simulink model "optimTRIAD"  (R2019a)
settings: Solver=VariableStepAuto  StartTime=0.0  StopTime=10.0  RelTol=1e-3
libraries: vrlib x8, dspstat3 x2, sharedtransform x1, aerolibutil x1
settings Model: Creator=Owner  LastModifiedBy=Owner

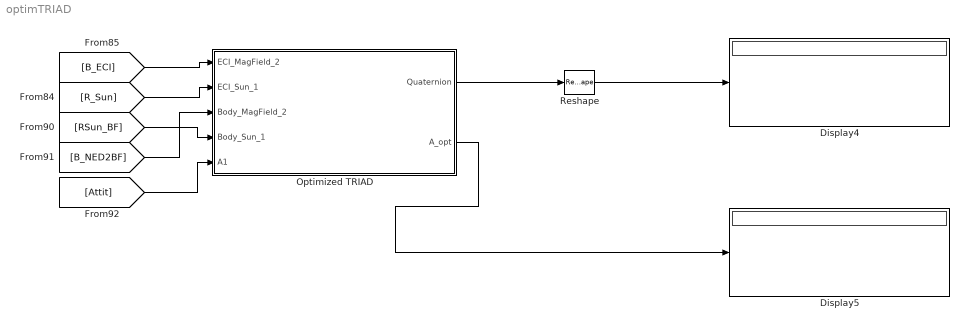
== system optimTRIAD ==
  Display4 : Display
  Display5 : Display
  "Optimized TRIAD " : Subsystem
  Reshape : Reshape  OutputDimensionality=Column vector (2-D)
  wires:
  [RSun_BF] -> "Optimized TRIAD "/4(Body_Sun_1)
  [Attit] -> "Optimized TRIAD "/5(A1)
  [B_NED2BF] -> "Optimized TRIAD "/3(Body_MagField_2)
  "Optimized TRIAD "/1(Quaternion) -> Reshape/1
  [B_ECI] -> "Optimized TRIAD "/1(ECI_MagField_2)
  [R_Sun] -> "Optimized TRIAD "/2(ECI_Sun_1)
  "Optimized TRIAD "/2(A_opt) -> Display5/1
  Reshape/1 -> Display4/1

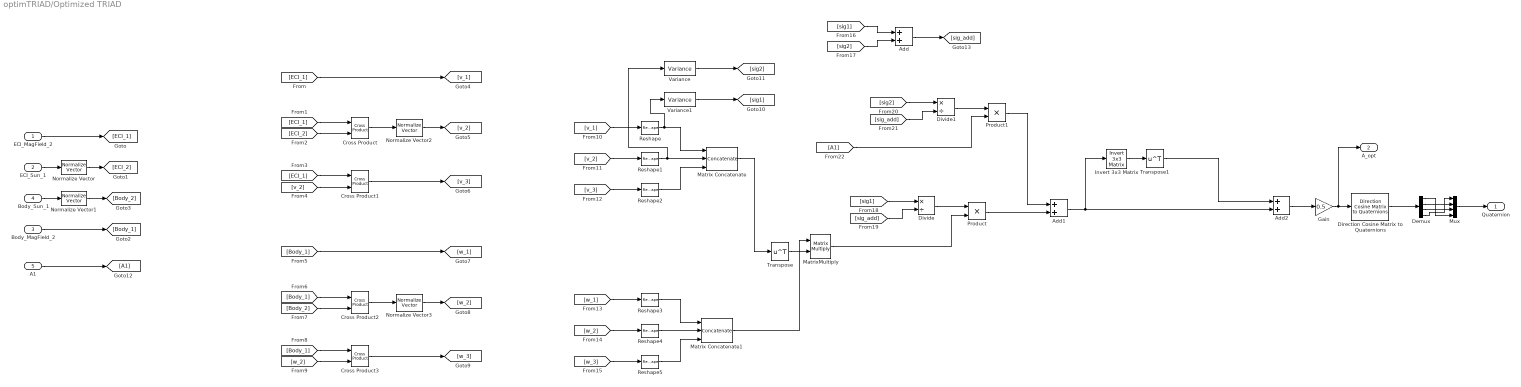
== system optimTRIAD/Optimized TRIAD  ==
  ECI_MagField_2 : Inport
  ECI_Sun_1 : Inport  Port=2
  Body_MagField_2 : Inport  Port=3
  Body_Sun_1 : Inport  Port=4
  A1 : Inport  Port=5
  Add : Sum
  Add1 : Sum
  Add2 : Sum
  Cross Product{,1..3} (4 alike) : vrlib/Utilities/Cross Product
  Demux : Demux
  Direction Cosine Matrix to Quaternions : sharedtransform/Direction Cosine Matrix  to Quaternions  aMode=0  action=None  tolerance=eps(2)
      settings: SourceProductBaseCode=AE,PW,MT,UV,VE,VP
  Divide : Product  Inputs=*/
  Divide1 : Product  Inputs=*/
  Gain : Gain  Gain=0.5
  Invert 3x3 Matrix : aerolibutil/Invert  3x3 Matrix
  Matrix Concatenate : Concatenate  NumInputs=3  Mode=Multidimensional array  ConcatenateDimension=2
  Matrix Concatenate1 : Concatenate  NumInputs=3  Mode=Multidimensional array  ConcatenateDimension=2
  MatrixMultiply : Product  Multiplication=Matrix(*)
  Mux : Mux
  Normalize Vector{,1..3} (4 alike) : vrlib/Utilities/Normalize Vector  maxzero=0
  Product : Product
  Product1 : Product
  Reshape{,1..5} (6 alike) : Reshape  OutputDimensionality=Column vector (2-D)
  Transpose : Math  Operator=transpose  SaturateOnIntegerOverflow=on
  Transpose1 : Math  Operator=transpose  SaturateOnIntegerOverflow=on
  Variance : dspstat3/Variance  run=off  InputProcessing=Columns as channels (frame based)  reset_popup=None  directionMode=Each column  dimension=1  roiEnable=off  roiType=Rectangles  roiPortion=Entire ROI  roiOutput=Individual statistics for each ROI  roiFlag=off  roundingMode=Floor  overflowMode=off
      settings: SourceProductName=DSP System Toolbox
  Variance1 : dspstat3/Variance  run=off  InputProcessing=Columns as channels (frame based)  reset_popup=None  directionMode=Each column  dimension=1  roiEnable=off  roiType=Rectangles  roiPortion=Entire ROI  roiOutput=Individual statistics for each ROI  roiFlag=off  roundingMode=Floor  overflowMode=off
      settings: SourceProductName=DSP System Toolbox
  Quaternion : Outport  VectorParamsAs1DForOutWhenUnconnected=on
  A_opt : Outport  Port=2  VectorParamsAs1DForOutWhenUnconnected=on
  wires:
  Cross Product/1 -> Normalize Vector2/1
  [ECI_1] -> Cross Product1/1
  Reshape2/1 -> Matrix Concatenate/3
  Cross Product3/1 -> [w_3]
  [ECI_1] -> [v_1]
  [w_1] -> Reshape3/1
  Body_Sun_1/1 -> Normalize Vector1/1
  [Body_1] -> Cross Product2/1
  [ECI_1] -> Cross Product/1
  Normalize Vector3/1 -> [w_2]
  Cross Product2/1 -> Normalize Vector3/1
  [Body_1] -> Cross Product3/1
  Cross Product1/1 -> [v_3]
  Normalize Vector2/1 -> [v_2]
  [ECI_2] -> Cross Product/2
  Reshape3/1 -> Matrix Concatenate1/1
  [v_2] -> Cross Product1/2
  [Body_1] -> [w_1]
  [w_3] -> Reshape5/1
  [v_3] -> Reshape2/1
  [v_1] -> Reshape/1
  [w_2] -> Cross Product3/2
  [Body_2] -> Cross Product2/2
  [w_2] -> Reshape4/1
  Reshape5/1 -> Matrix Concatenate1/3
  Reshape/1 -> Variance1/1, Matrix Concatenate/1
  Reshape4/1 -> Matrix Concatenate1/2
  Matrix Concatenate1/1 -> MatrixMultiply/1
  Matrix Concatenate/1 -> Transpose/1
  Transpose/1 -> MatrixMultiply/2
  Direction Cosine Matrix to Quaternions/1 -> Demux/1
  Demux/1 -> Mux/4
  Demux/2 -> Mux/1
  Demux/3 -> Mux/2
  Demux/4 -> Mux/3
  Mux/1 -> Quaternion/1
  [v_2] -> Reshape1/1
  Variance1/1 -> [sig1]
  Variance/1 -> [sig2]
  Reshape1/1 -> Variance/1, Matrix Concatenate/2
  ECI_MagField_2/1 -> [ECI_1]
  ECI_Sun_1/1 -> Normalize Vector/1
  Normalize Vector/1 -> [ECI_2]
  Body_MagField_2/1 -> [Body_1]
  Normalize Vector1/1 -> [Body_2]
  A1/1 -> [A1]
  [sig1] -> Add/1
  [sig2] -> Add/2
  Add/1 -> [sig_add]
  [sig1] -> Divide/1
  [sig_add] -> Divide/2
  Divide/1 -> Product/1
  MatrixMultiply/1 -> Product/2
  Product/1 -> Add1/2
  [A1] -> Product1/2
  [sig_add] -> Divide1/2
  [sig2] -> Divide1/1
  Divide1/1 -> Product1/1
  Product1/1 -> Add1/1
  Add1/1 -> Invert 3x3 Matrix/1, Add2/2
  Invert 3x3 Matrix/1 -> Transpose1/1
  Transpose1/1 -> Add2/1
  Add2/1 -> Gain/1
  Gain/1 -> A_opt/1, Direction Cosine Matrix to Quaternions/1
